simulink model "HILModel"  (Simulink 6.6)
settings: Solver=ode4  StartTime=0.0  StopTime=inf  FixedStep=SampleT  RelTol=1e-3
InitFcn:
  | clc
  | hilInit
values from neighbouring files (symbols this model uses):
  Euler_0 = [0; 0; 0*pi/180]'    [hilInit.m]
  HIL_K = 3    [hilInit.m]
  Pos_0 = [200; 350; 350]'    [hilInit.m]
  SampleT = 0.005    [hilInit.m]
  windBase = 3.5    [hilInit.m]
undefined symbols (not defined in the file or in its folder): A1, Apolar, bPWMda, bPWMde, bPWMdr, bPWMdt, CD0, chord, CL0, CLa, CLa_dot, Clb, ClDa, CLDe, CLDf, ClDr, clock, Clp, CLq, Clr, Cm0, Cma, CmDe, CmDf, Cmq, Cnb, CnDa, CnDr, Cnp, Cnr, CYb, CYDr, da_failamp, da_failbias, da_failper, daL_fail, daR_fail, DiscIntNeverNeededParam, dr_fail, Earth, elarm, F, GS_location, ISA_g, Ixx, Iyy, Izz, Light, mass, MIL, MinThK, mPWMda, mPWMde, mPWMdr, mPWMdt, PQR_0, span, tfailure, ThK, Vb_0 ... (+1)
libraries: simulink x31, aerolibconvert2 x8, xpclib x8, aerolibactuator x5, aerolibtransform2 x2, aerolibwind2 x2, dspmtrx3 x2, aerolibnav x2, aerolibatmos2 x1, aerolibanimutils x1
(part 1 of 2)
CloseFcn:
  | rtwprivate ssgencode ModelCloseRequest AttitudeComplementary
settings Model: Creator=ASL_Lab  LastModifiedBy=Administrator
settings DebuggingCC: AlgebraicLoopMsg=error  MultiTaskDSMMsg=warning  MultiTaskCondExecSysMsg=none  StrictBusMsg=None
settings HardwareCC: TargetHWDeviceType=32-bit Generic
settings RTWCC: IncludeERTFirstTime=on

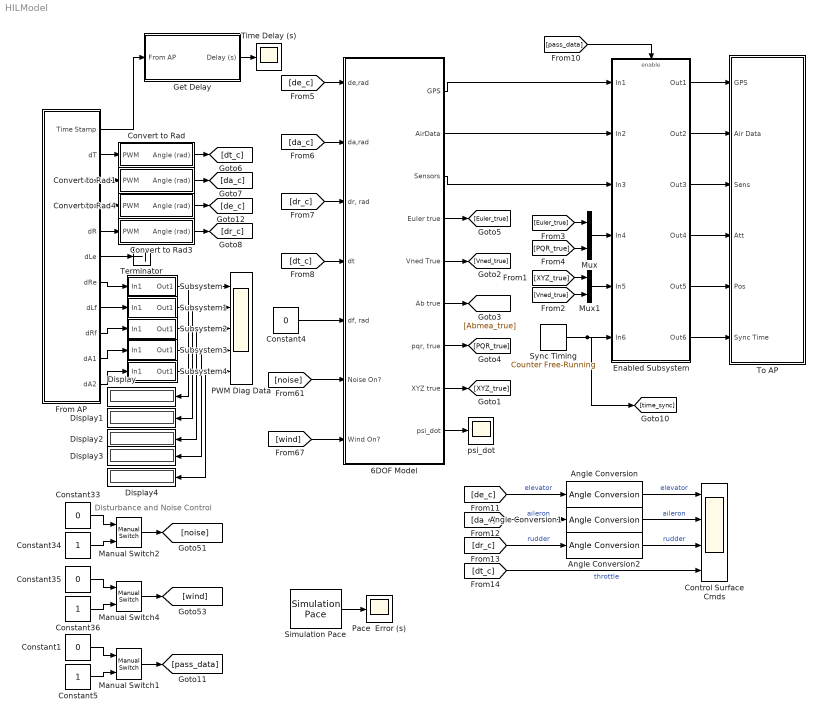
== system HILModel ==
  note: Disturbance and Noise Control
  6DOF Model : Subsystem
  Angle Conversion : aerolibconvert2/Angle Conversion  SystemSampleTime=-1  IU=rad  OU=deg
  Angle Conversion1 : aerolibconvert2/Angle Conversion  SystemSampleTime=-1  IU=rad  OU=deg
  Angle Conversion2 : aerolibconvert2/Angle Conversion  SystemSampleTime=-1  IU=rad  OU=deg
  Constant1 : Constant  Value=0  SampleTime=SampleT
  Constant33 : Constant  Value=0  SampleTime=SampleT
  Constant34 : Constant  SampleTime=SampleT
  Constant35 : Constant  Value=0  SampleTime=SampleT
  Constant36 : Constant  SampleTime=SampleT
  Constant4 : Constant  Value=0
  Constant5 : Constant  SampleTime=SampleT
  Control Surface Cmds : Scope  NumInputPorts=4
      settings: TimeRange=70  YMin=-55~-65~-75~-2.5  YMax=10~15~5~1  MaxDataPoints=25000
  Convert to Rad : Subsystem  mask{slopem=mPWMdt, interceptb=bPWMdt}
      mask prompts: slopem "Slope"; interceptb "Intercept"
  Convert to Rad1 : Subsystem  mask{slopem=mPWMda, interceptb=bPWMda}
      mask prompts: slopem "Slope"; interceptb "Intercept"
  Convert to Rad3 : Subsystem  mask{slopem=mPWMdr, interceptb=bPWMdr}
      mask prompts: slopem "Slope"; interceptb "Intercept"
  Convert to Rad4 : Subsystem  mask{slopem=mPWMde, interceptb=bPWMde}
      mask prompts: slopem "Slope"; interceptb "Intercept"
  Display{,1..4} (5 alike) : Display
  Enabled Subsystem : Subsystem  TreatAsAtomicUnit=on
  From AP : Subsystem
  Get Delay : Subsystem
  Manual Switch1 : simulink/Signal Routing/Manual Switch  SystemSampleTime=-1  sw=0  action=0  varsize=off
  Manual Switch2 : simulink/Signal Routing/Manual Switch  SystemSampleTime=-1  sw=1  action=0  varsize=off
  Manual Switch4 : simulink/Signal Routing/Manual Switch  SystemSampleTime=-1  sw=1  action=0  varsize=off
  Mux : Mux  Inputs=2
  Mux1 : Mux  Inputs=2
  PWM Diag Data : Scope  NumInputPorts=5
      settings: TimeRange=54.25925925925927  YMin=-31500~-33000~-34406.4~-34406.4~-35000  YMax=-28750~-28500~-31129.6~-31129.6~-15000  SaveName=ScopeData5  MaxDataPoints=25000
  Pace  Error (s) : Scope
      settings: YMin=-0.01  YMax=0.015  MaxDataPoints=25000
  Simulation Pace : aerolibanimutils/Simulation Pace  SimulationPace=1  SleepMode=MATLAB Thread  OutputPaceError=on  SampleTime=SampleT
      settings: AttributesFormatString=%<SimulationPace> sec/sec
  Subsystem : Subsystem
  Subsystem1 : Subsystem
  Subsystem2 : Subsystem
  Subsystem3 : Subsystem
  Subsystem4 : Subsystem
  Sync Timing : simulink/Sources/Counter Free-Running  SystemSampleTime=-1  NumBits=16  tsamp=SampleT
  Terminator : Terminator
  Time Delay (s) : Scope
      settings: TimeRange=60  YMin=0  YMax=0.05  SaveName=ScopeData2
  To AP : Subsystem
  psi_dot : Scope
      settings: TimeRange=120  YMin=-0.4  YMax=0.3  SaveName=ScopeData3  MaxDataPoints=25000
  wires:
  [PQR_true] -> Mux/2
  [XYZ_true] -> Mux1/1
  [Vned_true] -> Mux1/2
  [Euler_true] -> Mux/1
  Enabled Subsystem/1(Out1) -> To AP/1(GPS)
  Enabled Subsystem/2(Out2) -> To AP/2(Air Data)
  Enabled Subsystem/3(Out3) -> To AP/3(Sens)
  Enabled Subsystem/4(Out4) -> To AP/4(Att)
  Enabled Subsystem/5(Out5) -> To AP/5(Pos)
  Enabled Subsystem/6(Out6) -> To AP/6(Sync Time)
  6DOF Model/1(GPS) -> Enabled Subsystem/1(In1)
  6DOF Model/2(AirData) -> Enabled Subsystem/2(In2)
  6DOF Model/3(Sensors) -> Enabled Subsystem/3(In3)
  Mux/1 -> Enabled Subsystem/4(In4)
  Mux1/1 -> Enabled Subsystem/5(In5)
  Sync Timing/1 -> Enabled Subsystem/6(In6), [time_sync]
  6DOF Model/4(Euler true) -> [Euler_true]
  6DOF Model/5(Vned True) -> [Vned_true]
  6DOF Model/6(Ab true) -> [Abmea_true]
  6DOF Model/7("pqr, true") -> [PQR_true]
  6DOF Model/8(XYZ true) -> [XYZ_true]
  Constant4/1 -> 6DOF Model/5("df, rad")
  Constant33/1 -> Manual Switch2/1
  Constant34/1 -> Manual Switch2/2
  Manual Switch2/1 -> [noise]
  Constant35/1 -> Manual Switch4/1
  Constant36/1 -> Manual Switch4/2
  Manual Switch4/1 -> [wind]
  [noise] -> 6DOF Model/6(Noise On?)
  [wind] -> 6DOF Model/7(Wind On?)
  Constant1/1 -> Manual Switch1/1
  Constant5/1 -> Manual Switch1/2
  Manual Switch1/1 -> [pass_data]
  [pass_data] -> Enabled Subsystem/Enable
  From AP/3(dLa) -> Convert to Rad1/1(PWM)
  From AP/5(dR) -> Convert to Rad3/1(PWM)
  From AP/2(dT) -> Convert to Rad/1(PWM)
  From AP/4(dRa) -> Convert to Rad4/1(PWM)
  Get Delay/1(Delay (s)) -> Time Delay (s)/1
  From AP/1(Time Stamp) -> Get Delay/1(From AP)
  Convert to Rad/1(Angle (rad)) -> [dt_c]
  Convert to Rad1/1(Angle (rad)) -> [da_c]
  Convert to Rad3/1(Angle (rad)) -> [dr_c]
  From AP/6(dLe) -> Terminator/1
  [de_c] -> Angle Conversion/1  "elevator"
  [da_c] -> Angle Conversion1/1  "aileron"
  [dr_c] -> Angle Conversion2/1  "rudder"
  [dt_c] -> Control Surface Cmds/4  "throttle"
  [de_c] -> 6DOF Model/1(de,rad)
  [dt_c] -> 6DOF Model/4(dt)
  [dr_c] -> 6DOF Model/3("dr, rad")
  [da_c] -> 6DOF Model/2(da,rad)
  Angle Conversion/1 -> Control Surface Cmds/1  "elevator"
  Angle Conversion1/1 -> Control Surface Cmds/2  "aileron"
  Angle Conversion2/1 -> Control Surface Cmds/3  "rudder"
  Simulation Pace/1 -> Pace  Error (s)/1
  6DOF Model/9(psi_dot) -> psi_dot/1
  Subsystem/1(Out1) -> Display/1, PWM Diag Data/1
  Subsystem1/1(Out1) -> PWM Diag Data/2, Display1/1
  Subsystem2/1(Out1) -> PWM Diag Data/3, Display2/1
  Subsystem3/1(Out1) -> PWM Diag Data/4, Display3/1
  Subsystem4/1(Out1) -> PWM Diag Data/5, Display4/1
  From AP/7(dRe) -> Subsystem/1(In1)
  From AP/8(dLf) -> Subsystem1/1(In1)
  From AP/9(dRf) -> Subsystem2/1(In1)
  From AP/10(dA1) -> Subsystem3/1(In1)
  From AP/11(dA2) -> Subsystem4/1(In1)
  Convert to Rad4/1(Angle (rad)) -> [de_c]

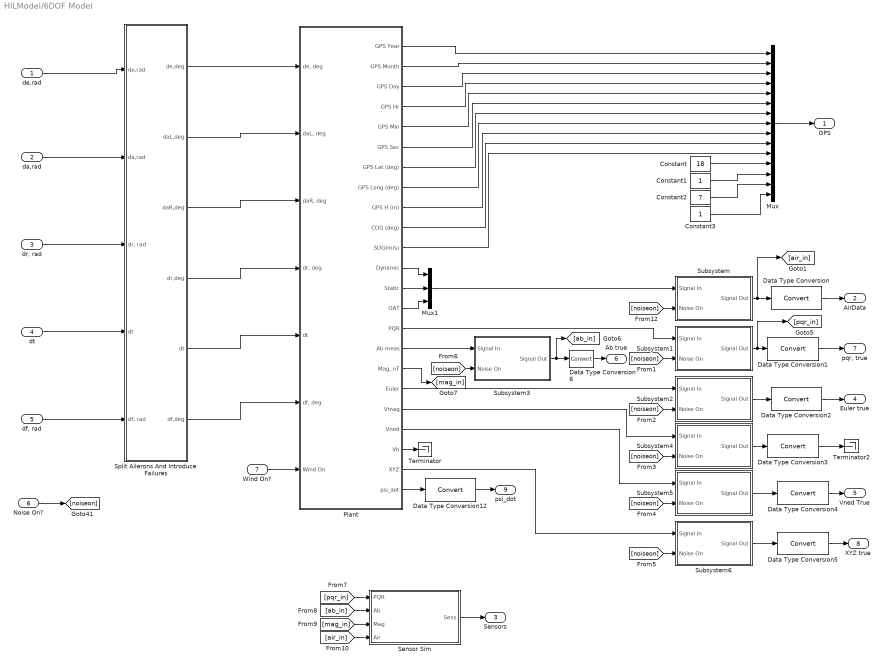
== system HILModel/6DOF Model ==
  de,rad : Inport
  da,rad : Inport  Port=2
  "dr, rad" : Inport  Port=3
  dt : Inport  Port=4
  "df, rad" : Inport  Port=5
  Noise On? : Inport  Port=6
  Wind On? : Inport  Port=7
  Constant : Constant  Value=18  SampleTime=SampleT
  Constant1 : Constant  SampleTime=SampleT
  Constant2 : Constant  Value=7  SampleTime=SampleT
  Constant3 : Constant  SampleTime=SampleT
  Data Type Conversion{,1..6,12} (8 alike) : DataTypeConversion  OutDataTypeMode=single
  Mux : Mux  Inputs=15
  Mux1 : Mux  Inputs=3
  Plant : Subsystem
  Sensor Sim : Subsystem
  Split Ailerons And Introduce Failures : Subsystem
  Subsystem : Subsystem  mask{nv=[0.01 0.01 0.1], st=SampleT, ns=[132 564 987]}
      mask prompts: nv "Noise Variance"; st "Sample Time"; ns "Noise Seed"
  Subsystem1 : Subsystem  mask{nv=[0.001 0.001 0.001], st=SampleT, ns=[132 564 987]}
      mask prompts: nv "Noise Variance"; st "Sample Time"; ns "Noise Seed"
  Subsystem2 : Subsystem  mask{nv=[0.0001 0.00003 0.0001], st=SampleT, ns=[132 564 987]}
      mask prompts: nv "Noise Variance"; st "Sample Time"; ns "Noise Seed"
  Subsystem3 : Subsystem  mask{nv=[0.1 0.1 0.1], st=SampleT, ns=[132 564 987]}
      mask prompts: nv "Noise Variance"; st "Sample Time"; ns "Noise Seed"
  Subsystem4 : Subsystem  mask{nv=[0.01], st=SampleT, ns=[321564]}
      mask prompts: nv "Noise Variance"; st "Sample Time"; ns "Noise Seed"
  Subsystem5 : Subsystem  mask{nv=[0.01 0.01 0.01], st=SampleT, ns=[321564 6546 98798]}
      mask prompts: nv "Noise Variance"; st "Sample Time"; ns "Noise Seed"
  Subsystem6 : Subsystem  mask{nv=[0.05 0.05 0.07], st=SampleT, ns=[321564]}
      mask prompts: nv "Noise Variance"; st "Sample Time"; ns "Noise Seed"
  Terminator : Terminator
  Terminator2 : Terminator
  GPS : Outport
  AirData : Outport  Port=2
  Sensors : Outport  Port=3
  Euler true : Outport  Port=4
  Vned True : Outport  Port=5
  Ab true : Outport  Port=6
  "pqr, true" : Outport  Port=7
  XYZ true : Outport  Port=8
  psi_dot : Outport  Port=9
  wires:
  Data Type Conversion12/1 -> psi_dot/1
  Data Type Conversion6/1 -> Ab true/1
  Data Type Conversion5/1 -> XYZ true/1
  Data Type Conversion4/1 -> Vned True/1
  Data Type Conversion3/1 -> Terminator2/1
  Data Type Conversion2/1 -> Euler true/1
  Data Type Conversion1/1 -> "pqr, true"/1
  Data Type Conversion/1 -> AirData/1
  Wind On?/1 -> Plant/7(Wind On)
  Plant/17("Mag, nT") -> [mag_in]
  Plant/21(Vb) -> Terminator/1
  Plant/22(XYZ) -> Subsystem6/1(Signal In)
  Subsystem6/1(Signal Out) -> Data Type Conversion5/1
  Plant/20(Vned) -> Subsystem5/1(Signal In)
  Subsystem5/1(Signal Out) -> Data Type Conversion4/1
  Plant/19(Vmag) -> Subsystem4/1(Signal In)
  Subsystem4/1(Signal Out) -> Data Type Conversion3/1
  Plant/16(Ab meas) -> Subsystem3/1(Signal In)
  Subsystem3/1(Signal Out) -> Data Type Conversion6/1, [ab_in]
  Plant/18(Euler) -> Subsystem2/1(Signal In)
  Subsystem2/1(Signal Out) -> Data Type Conversion2/1
  Plant/15(PQR) -> Subsystem1/1(Signal In)
  Subsystem1/1(Signal Out) -> Data Type Conversion1/1, [pqr_in]
  [noiseon] -> Subsystem3/2(Noise On)
  [noiseon] -> Subsystem6/2(Noise On)
  [noiseon] -> Subsystem5/2(Noise On)
  [noiseon] -> Subsystem4/2(Noise On)
  [noiseon] -> Subsystem2/2(Noise On)
  [noiseon] -> Subsystem1/2(Noise On)
  [noiseon] -> Subsystem/2(Noise On)
  Subsystem/1(Signal Out) -> Data Type Conversion/1, [air_in]
  Noise On?/1 -> [noiseon]
  Plant/23(psi_dot) -> Data Type Conversion12/1
  Constant3/1 -> Mux/15
  Constant2/1 -> Mux/14
  Constant1/1 -> Mux/13
  Constant/1 -> Mux/12
  Mux1/1 -> Subsystem/1(Signal In)
  Plant/14(OAT) -> Mux1/3
  Plant/13(Static) -> Mux1/2
  Plant/12(Dynamic) -> Mux1/1
  Plant/11(SOG(m/s)) -> Mux/11
  Plant/10(COG (deg)) -> Mux/10
  Plant/9(GPS H (m)) -> Mux/9
  Plant/8(GPS Long (deg)) -> Mux/8
  Plant/7(GPS Lat (deg)) -> Mux/7
  Plant/6(GPS Sec) -> Mux/6
  Plant/5(GPS Min) -> Mux/5
  Plant/4(GPS Hr) -> Mux/4
  Plant/3(GPS Day) -> Mux/3
  Plant/2(GPS Month) -> Mux/2
  Plant/1(GPS Year) -> Mux/1
  Mux/1 -> GPS/1
  "df, rad"/1 -> Split Ailerons And Introduce Failures/5("df, rad")
  dt/1 -> Split Ailerons And Introduce Failures/4(dt)
  "dr, rad"/1 -> Split Ailerons And Introduce Failures/3("dr, rad")
  da,rad/1 -> Split Ailerons And Introduce Failures/2(da,rad)
  de,rad/1 -> Split Ailerons And Introduce Failures/1(de,rad)
  Sensor Sim/1(Sens) -> Sensors/1
  [pqr_in] -> Sensor Sim/1(PQR)
  [ab_in] -> Sensor Sim/2(Ab)
  [mag_in] -> Sensor Sim/3(Mag)
  Split Ailerons And Introduce Failures/1(de,deg) -> Plant/1("de, deg")
  Split Ailerons And Introduce Failures/2(daL,deg) -> Plant/2("daL, deg")
  Split Ailerons And Introduce Failures/3(daR,deg) -> Plant/3("daR, deg")
  Split Ailerons And Introduce Failures/4(dr,deg) -> Plant/4("dr, deg")
  Split Ailerons And Introduce Failures/5("dt ") -> Plant/5(dt)
  Split Ailerons And Introduce Failures/6(df,deg) -> Plant/6("df, deg")
  [air_in] -> Sensor Sim/4(Air)

== system HILModel/Convert to Rad ==
  PWM : Inport  Orientation=down
  Add : Sum  OutScaling=2^-10
  Constant1 : Constant  Value=slopem
  Constant2 : Constant  Value=interceptb
  Data Type Conversion : DataTypeConversion  OutDataTypeMode=single
  Divide : Product  OutScaling=2^-10
  Angle (rad) : Outport
  wires:
  Constant1/1 -> Divide/2
  Add/1 -> Data Type Conversion/1
  Divide/1 -> Add/1
  Constant2/1 -> Add/2
  PWM/1 -> Divide/1
  Data Type Conversion/1 -> Angle (rad)/1

== system HILModel/Convert to Rad1 ==
  PWM : Inport  Orientation=down
  Add : Sum  OutScaling=2^-10
  Constant1 : Constant  Value=slopem
  Constant2 : Constant  Value=interceptb
  Data Type Conversion : DataTypeConversion  OutDataTypeMode=single
  Divide : Product  OutScaling=2^-10
  Angle (rad) : Outport
  wires:
  Data Type Conversion/1 -> Angle (rad)/1
  PWM/1 -> Divide/1
  Constant2/1 -> Add/2
  Divide/1 -> Add/1
  Add/1 -> Data Type Conversion/1
  Constant1/1 -> Divide/2

== system HILModel/Convert to Rad3 ==
  PWM : Inport  Orientation=down
  Add : Sum  OutScaling=2^-10
  Constant1 : Constant  Value=slopem
  Constant2 : Constant  Value=interceptb
  Data Type Conversion : DataTypeConversion  OutDataTypeMode=single
  Divide : Product  OutScaling=2^-10
  Angle (rad) : Outport
  wires:
  Data Type Conversion/1 -> Angle (rad)/1
  PWM/1 -> Divide/1
  Constant2/1 -> Add/2
  Divide/1 -> Add/1
  Add/1 -> Data Type Conversion/1
  Constant1/1 -> Divide/2

== system HILModel/Convert to Rad4 ==
  PWM : Inport  Orientation=down
  Add : Sum  OutScaling=2^-10
  Constant1 : Constant  Value=slopem
  Constant2 : Constant  Value=interceptb
  Data Type Conversion : DataTypeConversion  OutDataTypeMode=single
  Divide : Product  OutScaling=2^-10
  Angle (rad) : Outport
  wires:
  Data Type Conversion/1 -> Angle (rad)/1
  PWM/1 -> Divide/1
  Constant2/1 -> Add/2
  Divide/1 -> Add/1
  Add/1 -> Data Type Conversion/1
  Constant1/1 -> Divide/2

== system HILModel/Enabled Subsystem ==
  In1 : Inport
  In2 : Inport  Port=2
  In3 : Inport  Port=3
  In4 : Inport  Port=4
  In5 : Inport  Port=5
  In6 : Inport  Port=6
  Enable : EnablePort
  Out1 : Outport
  Out2 : Outport  Port=2
  Out3 : Outport  Port=3
  Out4 : Outport  Port=4
  Out5 : Outport  Port=5
  Out6 : Outport  Port=6
  wires:
  In1/1 -> Out1/1
  In2/1 -> Out2/1
  In3/1 -> Out3/1
  In4/1 -> Out4/1
  In5/1 -> Out5/1
  In6/1 -> Out6/1

== system HILModel/From AP ==
  Bus Creator : BusCreator  Inputs=11
  Bus Selector : BusSelector  OutputSignals=dt,dla,dra,dr,dle,dre,dlf,drf,da1,da2,timeStamp
  Display : Display
  Receive : xpclib/UDP/Receive  ipAddress=0.0.0.0  ipPort=5678  width=22  sampletime=SampleT
  Terminator : Terminator
  Unpack1 : xpclib/UDP/Unpack  dimensions={1,1,1,1,1,1,1,1,1,1,1}  datatypes={'uint16','uint16','uint16','uint16', 'uint16', 'uint16','uint16', 'uint16','uint16', 'uint16','uint16'}  byteAlign=1
  Time Stamp : Outport
  dT : Outport  Port=2
  dLa : Outport  Port=3
  dRa : Outport  Port=4
  dR : Outport  Port=5
  dLe : Outport  Port=6
  dRe : Outport  Port=7
  dLf : Outport  Port=8
  dRf : Outport  Port=9
  dA1 : Outport  Port=10
  dA2 : Outport  Port=11
  wires:
  Receive/1 -> Unpack1/1
  Receive/2 -> Terminator/1
  Bus Creator/1 -> Bus Selector/1, Display/1
  Unpack1/1 -> Bus Creator/1  "dt"
  Unpack1/3 -> Bus Creator/3  "dra"
  Unpack1/5 -> Bus Creator/5  "dle"
  Unpack1/7 -> Bus Creator/7  "dlf"
  Unpack1/9 -> Bus Creator/9  "da1"
  Unpack1/11 -> Bus Creator/11  "timeStamp"
  Bus Selector/1 -> dT/1  "<dt>"
  Bus Selector/2 -> dLa/1  "<dla>"
  Bus Selector/3 -> dRa/1  "<dra>"
  Bus Selector/4 -> dR/1  "<dr>"
  Bus Selector/5 -> dLe/1  "<dle>"
  Bus Selector/6 -> dRe/1  "<dre>"
  Bus Selector/7 -> dLf/1  "<dlf>"
  Bus Selector/8 -> dRf/1  "<drf>"
  Bus Selector/9 -> dA1/1  "<da1>"
  Bus Selector/10 -> dA2/1  "<da2>"
  Bus Selector/11 -> Time Stamp/1  "<timeStamp>"
  Unpack1/2 -> Bus Creator/2  "dla"
  Unpack1/4 -> Bus Creator/4  "dr"
  Unpack1/6 -> Bus Creator/6  "dre"
  Unpack1/8 -> Bus Creator/8  "drf"
  Unpack1/10 -> Bus Creator/10  "da2"

== system HILModel/Get Delay ==
  From AP : Inport
  Detect Change : Subsystem
  GPSAlive : Subsystem
  Delay (s) : Outport
  wires:
  From AP/1 -> Detect Change/1(Data)
  Detect Change/1(change?) -> GPSAlive/1(update?)
  GPSAlive/1(Update TIme) -> Delay (s)/1

== system HILModel/Subsystem ==
  In1 : Inport
  Add : Sum  Inputs=+-  OutScaling=2^-10
  Constant : Constant  Value=32768
  Out1 : Outport
  wires:
  Constant/1 -> Add/2
  In1/1 -> Add/1
  Add/1 -> Out1/1

== system HILModel/Subsystem1 ==
  In1 : Inport
  Add : Sum  Inputs=+-  OutScaling=2^-10
  Constant : Constant  Value=32768
  Out1 : Outport
  wires:
  Add/1 -> Out1/1
  In1/1 -> Add/1
  Constant/1 -> Add/2

== system HILModel/Subsystem2 ==
  In1 : Inport
  Add : Sum  Inputs=+-  OutScaling=2^-10
  Constant : Constant  Value=32768
  Out1 : Outport
  wires:
  Constant/1 -> Add/2
  In1/1 -> Add/1
  Add/1 -> Out1/1

== system HILModel/Subsystem3 ==
  In1 : Inport
  Add : Sum  Inputs=+-  OutScaling=2^-10
  Constant : Constant  Value=32768
  Out1 : Outport
  wires:
  Add/1 -> Out1/1
  In1/1 -> Add/1
  Constant/1 -> Add/2

== system HILModel/Subsystem4 ==
  In1 : Inport
  Add : Sum  Inputs=+-  OutScaling=2^-10
  Constant : Constant  Value=32768
  Out1 : Outport
  wires:
  Constant/1 -> Add/2
  In1/1 -> Add/1
  Add/1 -> Out1/1

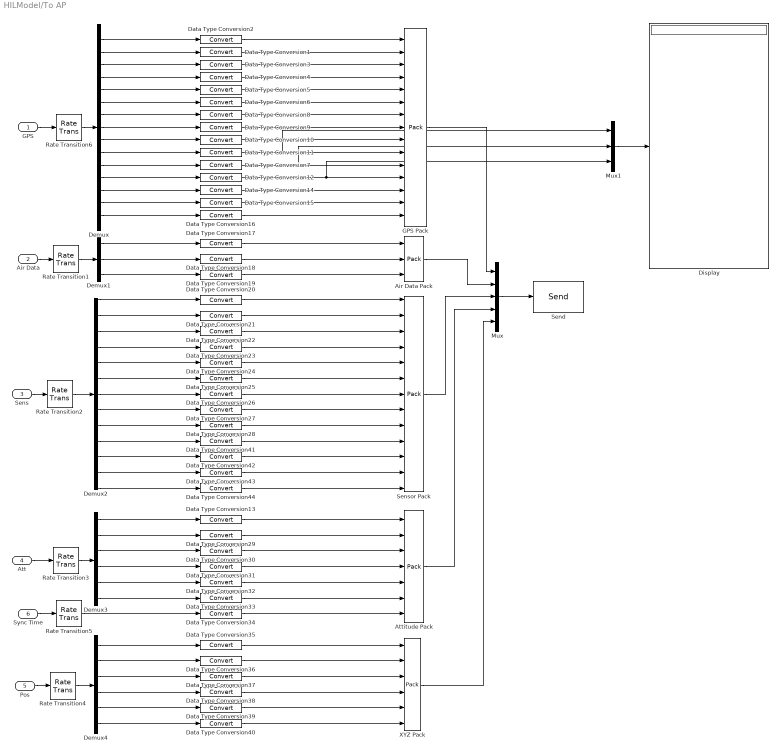
== system HILModel/To AP ==
  GPS : Inport
  Air Data : Inport  Port=2
  Sens : Inport  Port=3
  Att : Inport  Port=4
  Pos : Inport  Port=5
  Sync Time : Inport  Port=6
  Air Data Pack : xpclib/UDP/Pack  datatypes={'single', 'single', 'int16'}  byteAlign=1
  Attitude Pack : xpclib/UDP/Pack  datatypes={'single','single','single','single','single','single','uint16'}  byteAlign=1
  Data Type Conversion{1..6,14..16} (9 alike) : DataTypeConversion  OutDataTypeMode=uint8
  Data Type Conversion{8..10,13,17..18,29..33,35..40} (17 alike) : DataTypeConversion  OutDataTypeMode=single
  Data Type Conversion{7,11..12,34} (4 alike) : DataTypeConversion  OutDataTypeMode=uint16
  Data Type Conversion{19..28,41..44} (14 alike) : DataTypeConversion  OutDataTypeMode=int16
  Demux : Demux  Outputs=15
  Demux1 : Demux  Outputs=3
  Demux2 : Demux  Outputs=13
  Demux3 : Demux  Outputs=6
  Demux4 : Demux  Outputs=6
  Display : Display
  GPS Pack : xpclib/UDP/Pack  datatypes={'uint8','uint8','uint8','uint8','uint8','uint8', 'single', 'single', 'single', 'uint16', 'uint16', 'uint16', 'uint8', 'uint8', 'uint8'}  byteAlign=1
  Mux : Mux  Inputs=5
  Mux1 : Mux  Inputs=3
  Rate Transition{1..6} (6 alike) : RateTransition  OutPortSampleTime=SampleT*HIL_K
  Send : xpclib/UDP/Send  ipAddress=255.255.255.255  ipPort=5679  localPort=5678  sampletime=SampleT*HIL_K
  Sensor Pack : xpclib/UDP/Pack  datatypes={'int16', 'int16', 'int16', 'int16', 'int16', 'int16', 'int16', 'int16', 'int16', 'int16', 'int16', 'int16', 'int16'}  byteAlign=1
  XYZ Pack : xpclib/UDP/Pack  datatypes={'single','single','single','single','single','single'}  byteAlign=1
  wires:
  Demux/1 -> Data Type Conversion2/1
  Demux/2 -> Data Type Conversion1/1
  Demux/3 -> Data Type Conversion3/1
  Demux/4 -> Data Type Conversion4/1
  Demux/5 -> Data Type Conversion5/1
  Demux/6 -> Data Type Conversion6/1
  Demux/7 -> Data Type Conversion8/1
  Demux/8 -> Data Type Conversion9/1
  Demux/9 -> Data Type Conversion10/1
  Demux/10 -> Data Type Conversion11/1
  Demux/11 -> Data Type Conversion7/1
  Demux/12 -> Data Type Conversion12/1
  Demux/13 -> Data Type Conversion14/1
  Demux/14 -> Data Type Conversion15/1
  Demux/15 -> Data Type Conversion16/1
  Demux1/2 -> Data Type Conversion18/1
  Demux1/3 -> Data Type Conversion19/1
  Demux2/1 -> Data Type Conversion20/1
  Demux2/2 -> Data Type Conversion21/1
  Demux2/3 -> Data Type Conversion22/1
  Demux2/4 -> Data Type Conversion23/1
  Demux2/5 -> Data Type Conversion24/1
  Demux2/6 -> Data Type Conversion25/1
  Demux2/7 -> Data Type Conversion26/1
  Demux2/8 -> Data Type Conversion27/1
  Demux2/9 -> Data Type Conversion28/1
  Mux/1 -> Send/1
  GPS Pack/1 -> Mux/1
  Air Data Pack/1 -> Mux/2
  Sensor Pack/1 -> Mux/3
  GPS/1 -> Rate Transition6/1
  Air Data/1 -> Rate Transition1/1
  Sens/1 -> Rate Transition2/1
  Rate Transition6/1 -> Demux/1
  Rate Transition1/1 -> Demux1/1
  Rate Transition2/1 -> Demux2/1
  Att/1 -> Rate Transition3/1
  Pos/1 -> Rate Transition4/1
  Rate Transition3/1 -> Demux3/1
  Demux3/1 -> Data Type Conversion13/1
  Demux3/2 -> Data Type Conversion29/1
  Demux3/3 -> Data Type Conversion30/1
  Demux3/4 -> Data Type Conversion31/1
  Demux3/5 -> Data Type Conversion32/1
  Demux3/6 -> Data Type Conversion33/1
  Demux4/1 -> Data Type Conversion35/1
  Demux4/2 -> Data Type Conversion36/1
  Demux4/3 -> Data Type Conversion37/1
  Demux4/4 -> Data Type Conversion38/1
  Demux4/5 -> Data Type Conversion39/1
  Demux4/6 -> Data Type Conversion40/1
  Rate Transition4/1 -> Demux4/1
  Attitude Pack/1 -> Mux/4
  XYZ Pack/1 -> Mux/5
  Sync Time/1 -> Rate Transition5/1
  Data Type Conversion2/1 -> GPS Pack/1
  Data Type Conversion1/1 -> GPS Pack/2
  Data Type Conversion3/1 -> GPS Pack/3
  Data Type Conversion4/1 -> GPS Pack/4
  Data Type Conversion5/1 -> GPS Pack/5
  Data Type Conversion6/1 -> GPS Pack/6
  Data Type Conversion8/1 -> GPS Pack/7
  Data Type Conversion9/1 -> GPS Pack/8
  Data Type Conversion10/1 -> GPS Pack/9
  Data Type Conversion11/1 -> GPS Pack/10, Mux1/1
  Data Type Conversion7/1 -> GPS Pack/11, Mux1/2
  Data Type Conversion12/1 -> GPS Pack/12, Mux1/3
  Data Type Conversion14/1 -> GPS Pack/13
  Data Type Conversion15/1 -> GPS Pack/14
  Data Type Conversion16/1 -> GPS Pack/15
  Data Type Conversion17/1 -> Air Data Pack/1
  Data Type Conversion18/1 -> Air Data Pack/2
  Data Type Conversion19/1 -> Air Data Pack/3
  Data Type Conversion20/1 -> Sensor Pack/1
  Data Type Conversion21/1 -> Sensor Pack/2
  Data Type Conversion22/1 -> Sensor Pack/3
  Data Type Conversion23/1 -> Sensor Pack/4
  Data Type Conversion24/1 -> Sensor Pack/5
  Data Type Conversion25/1 -> Sensor Pack/6
  Data Type Conversion26/1 -> Sensor Pack/7
  Data Type Conversion27/1 -> Sensor Pack/8
  Data Type Conversion28/1 -> Sensor Pack/9
  Data Type Conversion13/1 -> Attitude Pack/1
  Data Type Conversion29/1 -> Attitude Pack/2
  Data Type Conversion30/1 -> Attitude Pack/3
  Data Type Conversion31/1 -> Attitude Pack/4
  Data Type Conversion32/1 -> Attitude Pack/5
  Data Type Conversion33/1 -> Attitude Pack/6
  Data Type Conversion34/1 -> Attitude Pack/7
  Data Type Conversion35/1 -> XYZ Pack/1
  Data Type Conversion36/1 -> XYZ Pack/2
  Data Type Conversion37/1 -> XYZ Pack/3
  Data Type Conversion38/1 -> XYZ Pack/4
  Data Type Conversion39/1 -> XYZ Pack/5
  Data Type Conversion40/1 -> XYZ Pack/6
  Demux1/1 -> Data Type Conversion17/1
  Rate Transition5/1 -> Data Type Conversion34/1
  Demux2/10 -> Data Type Conversion41/1
  Data Type Conversion41/1 -> Sensor Pack/10
  Demux2/11 -> Data Type Conversion42/1
  Data Type Conversion42/1 -> Sensor Pack/11
  Demux2/12 -> Data Type Conversion43/1
  Data Type Conversion43/1 -> Sensor Pack/12
  Demux2/13 -> Data Type Conversion44/1
  Data Type Conversion44/1 -> Sensor Pack/13
  Mux1/1 -> Display/1

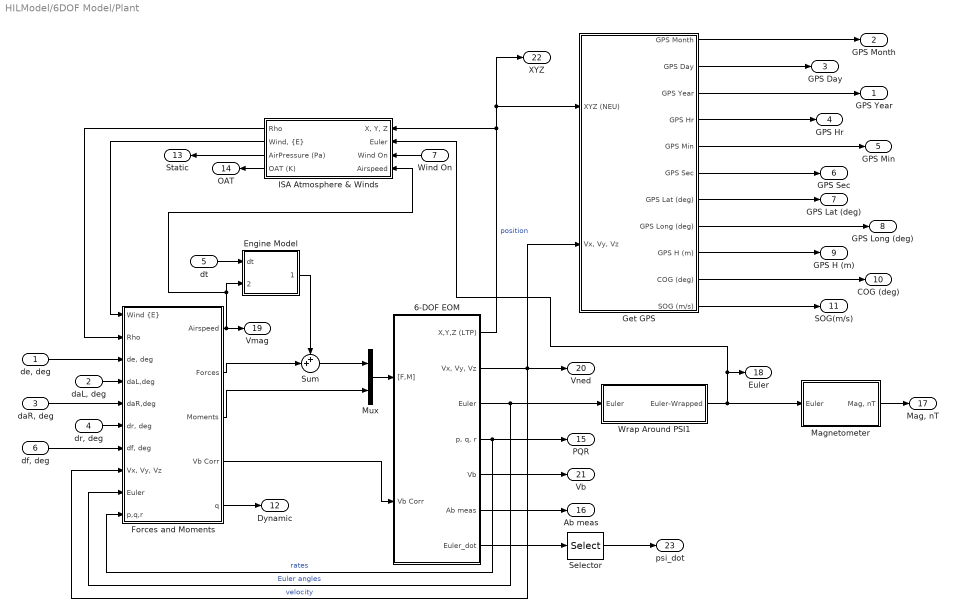
== system HILModel/6DOF Model/Plant ==
  "de, deg" : Inport
  "daL, deg" : Inport  Port=2
  "daR, deg" : Inport  Port=3
  "dr, deg" : Inport  Port=4
  dt : Inport  Port=5
  "df, deg" : Inport  Port=6
  Wind On : Inport  Orientation=left  Port=7
  6-DOF EOM : Subsystem
  Engine Model : Subsystem
  Forces and Moments : Subsystem
  Get GPS : Subsystem
  ISA Atmosphere & Winds : Subsystem  Orientation=left
  Magnetometer : Subsystem  mask{magField=[ 23143.6 5858.2 45511.9]}
      mask prompts: magField "Local Magnetic Field"
      mask help:
      | Simulates the Data from magnetometers with no noise.
      |
      | You can obtain data for the local magnetic field at:
      |
      | http://www.ngdc.noaa.gov/geomagmodels/IGRFWMM.jsp
  Mux : Mux  Inputs=2
  Selector : Selector  IndexOptions=Index vector (dialog)  Indices=[3]  OutputSizes=1  InputPortWidth=3
  Sum : Sum  Inputs=++|  SaturateOnIntegerOverflow=on
  Wrap Around PSI1 : Subsystem
  GPS Year : Outport
  GPS Month : Outport  Port=2
  GPS Day : Outport  Port=3
  GPS Hr : Outport  Port=4
  GPS Min : Outport  Port=5
  GPS Sec : Outport  Port=6
  GPS Lat (deg) : Outport  Port=7
  GPS Long (deg) : Outport  Port=8
  GPS H (m) : Outport  Port=9
  COG (deg) : Outport  Port=10
  SOG(m/s) : Outport  Port=11
  Dynamic : Outport  Port=12
  Static : Outport  Orientation=left  Port=13
  OAT : Outport  Orientation=left  Port=14
  PQR : Outport  Port=15
  Ab meas : Outport  Port=16
  "Mag, nT" : Outport  Port=17
  Euler : Outport  Port=18
  Vmag : Outport  Port=19
  Vned : Outport  Port=20
  Vb : Outport  Port=21
  XYZ : Outport  Port=22
  psi_dot : Outport  Port=23
  wires:
  Get GPS/1(GPS Month) -> GPS Month/1
  Get GPS/2(GPS Day) -> GPS Day/1
  Get GPS/3(GPS Year) -> GPS Year/1
  Get GPS/4(GPS Hr) -> GPS Hr/1
  Get GPS/5(GPS Min) -> GPS Min/1
  Get GPS/6(GPS Sec) -> GPS Sec/1
  Get GPS/7(GPS Lat (deg)) -> GPS Lat (deg)/1
  Get GPS/8(GPS Long (deg)) -> GPS Long (deg)/1
  Get GPS/9(GPS H (m)) -> GPS H (m)/1
  6-DOF EOM/6(Ab meas) -> Ab meas/1
  Mux/1 -> 6-DOF EOM/1("[F,M]")
  6-DOF EOM/5(Vb) -> Vb/1
  Engine Model/1(Thrust) -> Sum/1
  Forces and Moments/5(q) -> Dynamic/1
  ISA Atmosphere & Winds/3(AirPressure (Pa)) -> Static/1
  Forces and Moments/1(Airspeed) -> Vmag/1, Engine Model/2(Vmag), ISA Atmosphere & Winds/4(Airspeed)
  ISA Atmosphere & Winds/2("Wind, {E}") -> Forces and Moments/1("Wind {E}")
  ISA Atmosphere & Winds/1(Rho) -> Forces and Moments/2(Rho)
  Forces and Moments/3(Moments) -> Mux/2
  Forces and Moments/2(Forces) -> Sum/2
  Sum/1 -> Mux/1
  Forces and Moments/4(Vb Corr) -> 6-DOF EOM/2(Vb Corr)
  6-DOF EOM/1(X,Y,Z (LTP)) -> ISA Atmosphere & Winds/1("X, Y, Z"), Get GPS/1(XYZ (NEU)), XYZ/1  "position"
  6-DOF EOM/2("Vx, Vy, Vz") -> Vned/1, Get GPS/2("Vx, Vy, Vz"), Forces and Moments/8("Vx, Vy, Vz ")  "velocity"
  6-DOF EOM/3(Euler) -> Wrap Around PSI1/1(Euler), Forces and Moments/9(Euler)  "Euler angles"
  6-DOF EOM/4("p, q, r") -> PQR/1, Forces and Moments/10(p,q,r)  "rates"
  dt/1 -> Engine Model/1(dt)
  "de, deg"/1 -> Forces and Moments/3("de, deg")
  "daL, deg"/1 -> Forces and Moments/4(daL,deg)
  "dr, deg"/1 -> Forces and Moments/6("dr, deg")
  "df, deg"/1 -> Forces and Moments/7("df, deg")
  Wrap Around PSI1/1(Euler-Wrapped) -> Magnetometer/1(Euler), Euler/1, ISA Atmosphere & Winds/2(Euler)
  Magnetometer/1("Mag, nT") -> "Mag, nT"/1
  Get GPS/10(COG (deg)) -> COG (deg)/1
  Get GPS/11(SOG (m/s)) -> SOG(m/s)/1
  ISA Atmosphere & Winds/4(OAT (K)) -> OAT/1
  6-DOF EOM/7(Euler_dot) -> Selector/1
  Selector/1 -> psi_dot/1
  Wind On/1 -> ISA Atmosphere & Winds/3(Wind On)
  "daR, deg"/1 -> Forces and Moments/5(daR,deg)

== system HILModel/6DOF Model/Sensor Sim ==
  PQR : Inport
  Ab : Inport  Port=2
  Mag : Inport  Port=3
  Air : Inport  Port=4
  Constant : Constant  Value=2048
  Mux1 : Mux  Inputs=3
  Mux2 : Mux
  Selector : Selector  IndexOptions=Index vector (dialog)  Indices=[2 1]  OutputSizes=1  InputPortWidth=3
  Selector1 : Selector  IndexOptions=Index vector (dialog)  Indices=[3]  OutputSizes=1  InputPortWidth=3
  Three-axis Accelerometer : aerolibnav/Three-axis Accelerometer  SystemSampleTime=-1  units=Metric (MKS)  acc=[0 0 0]  gtype=off  dtype_a=on  w_a=190  z_a=0.707  a_sf_cc=[-41 0 0; 0 41 0; 0 0 -43]  a_bias=[2015 2018 2006]  a_rand=off  a_seeds=[23093 23094 23095]  a_pow=[0.008 0.008 0.008]  a_sat="[-inf  -inf  -inf  inf inf inf]"  a_Ts=SampleT
  Three-axis Gyroscope : aerolibnav/Three-axis Gyroscope  SystemSampleTime=-1  dtype_g=off  w_g=190  z_g=0.707  g_sf_cc=[-142 0 0; 0 142 0; 0 0 235]  g_bias=[1866 1981 2042]  g_sen=[0 0 0]  g_rand=off  g_seeds=[23093 23094 23095]  g_pow=[0.008 0.008 0.008]  g_sat="[-inf  -inf  -inf  inf inf inf]"  g_Ts=SampleT
  Sens : Outport
  wires:
  Mag/1 -> Mux2/3
  Mux2/1 -> Sens/1
  Ab/1 -> Three-axis Accelerometer/1
  PQR/1 -> Three-axis Gyroscope/1
  Three-axis Accelerometer/1 -> Mux2/2
  Three-axis Gyroscope/1 -> Mux2/1
  Air/1 -> Selector/1, Selector1/1
  Selector/1 -> Mux1/1
  Constant/1 -> Mux1/2
  Selector1/1 -> Mux1/3
  Mux1/1 -> Mux2/4

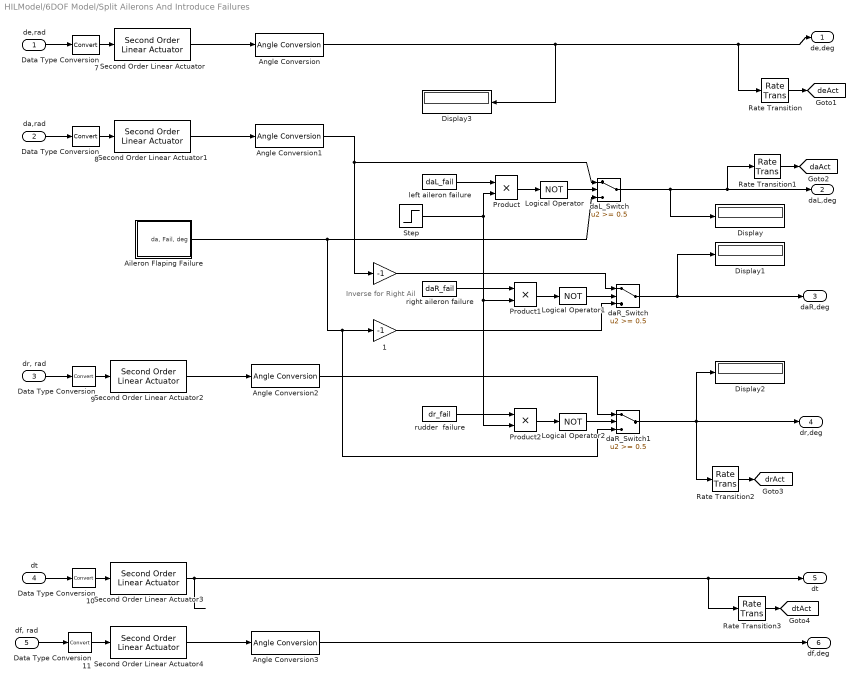
== system HILModel/6DOF Model/Split Ailerons And Introduce Failures ==
  note: Inverse
      | for Right
      | Ail
  de,rad : Inport
  da,rad : Inport  Port=2
  "dr, rad" : Inport  Port=3
  dt : Inport  Port=4
  "df, rad" : Inport  Port=5
  " " : Gain  Gain=-1  SaturateOnIntegerOverflow=on
  " 1" : Gain  Gain=-1  SaturateOnIntegerOverflow=on
  Aileron Flaping Failure : Subsystem
  Angle Conversion{,1..3} (4 alike) : aerolibconvert2/Angle Conversion  SystemSampleTime=-1  IU=rad  OU=deg
  Data Type Conversion{7..11} (5 alike) : DataTypeConversion  OutDataTypeMode=double
  Display{,1..3} (4 alike) : Display
  Logical Operator : Logic  Operator=NOT  AllPortsSameDT=off  OutDataTypeMode=Boolean
  Logical Operator1 : Logic  Operator=NOT  AllPortsSameDT=off  OutDataTypeMode=Boolean
  Logical Operator2 : Logic  Operator=NOT  AllPortsSameDT=off  OutDataTypeMode=Boolean
  Product : Product  RndMeth=Zero
  Product1 : Product  RndMeth=Zero
  Product2 : Product  RndMeth=Zero
  Rate Transition{,1..3} (4 alike) : RateTransition  OutPortSampleTime=apSampleTime
  Second Order Linear Actuator{,1..3} (4 alike) : aerolibactuator/Second Order Linear Actuator  SystemSampleTime=-1  wn_fin=15  z_fin=0.8  fin_act_0=0
  Second Order Linear Actuator4 : aerolibactuator/Second Order Linear Actuator  SystemSampleTime=-1  wn_fin=150  z_fin=0.7  fin_act_0=0
  Step : Step  Time=tfailure
  daL_Switch : Switch  Threshold=0.5
  daR_Switch : Switch  Threshold=0.5
  daR_Switch1 : Switch  Threshold=0.5
  left aileron failure : Constant  Value=daL_fail
  right aileron failure : Constant  Value=daR_fail
  rudder  failure : Constant  Value=dr_fail
  de,deg : Outport
  daL,deg : Outport  Port=2
  daR,deg : Outport  Port=3
  dr,deg : Outport  Port=4
  "dt " : Outport  Port=5
  df,deg : Outport  Port=6
  tag scope: daAct=global, deAct=global, drAct=global, dtAct=global
  wires:
  Rate Transition/1 -> [deAct]
  daR_Switch1/1 -> Rate Transition2/1, Display2/1, dr,deg/1
  Logical Operator2/1 -> daR_Switch1/2
  Product2/1 -> Logical Operator2/1
  rudder  failure/1 -> Product2/1
  daR_Switch/1 -> Display1/1, daR,deg/1
  " 1"/1 -> daR_Switch/3
  " "/1 -> daR_Switch/1
  Logical Operator1/1 -> daR_Switch/2
  Product1/1 -> Logical Operator1/1
  right aileron failure/1 -> Product1/1
  daL_Switch/1 -> Rate Transition1/1, daL,deg/1, Display/1
  Step/1 -> Product2/2, Product1/2, Product/2
  Logical Operator/1 -> daL_Switch/2
  Product/1 -> Logical Operator/1
  Aileron Flaping Failure/1("da, Fail, deg") -> daR_Switch1/3, " 1"/1, daL_Switch/3
  left aileron failure/1 -> Product/1
  Angle Conversion3/1 -> df,deg/1
  Angle Conversion2/1 -> daR_Switch1/1
  Angle Conversion1/1 -> " "/1, daL_Switch/1
  Angle Conversion/1 -> Rate Transition/1, de,deg/1, Display3/1
  Data Type Conversion11/1 -> Second Order Linear Actuator4/1
  Data Type Conversion10/1 -> Second Order Linear Actuator3/1
  Data Type Conversion9/1 -> Second Order Linear Actuator2/1
  Data Type Conversion8/1 -> Second Order Linear Actuator1/1
  Data Type Conversion7/1 -> Second Order Linear Actuator/1
  Rate Transition3/1 -> [dtAct]
  Rate Transition2/1 -> [drAct]
  Rate Transition1/1 -> [daAct]
  Second Order Linear Actuator4/1 -> Angle Conversion3/1
  Second Order Linear Actuator3/1 -> Rate Transition3/1, "dt "/1
  Second Order Linear Actuator2/1 -> Angle Conversion2/1
  Second Order Linear Actuator1/1 -> Angle Conversion1/1
  Second Order Linear Actuator/1 -> Angle Conversion/1
  "df, rad"/1 -> Data Type Conversion11/1
  dt/1 -> Data Type Conversion10/1
  "dr, rad"/1 -> Data Type Conversion9/1
  da,rad/1 -> Data Type Conversion8/1
  de,rad/1 -> Data Type Conversion7/1

== system HILModel/6DOF Model/Subsystem ==
  Signal In : Inport  Orientation=down
  Noise On : Inport  Port=2
  Add : Sum  OutScaling=2^-10
  Random Number : RandomNumber  Variance=nv  Seed=ns  SampleTime=st
  Signal1 : InportShadow  Port=1  LatchByCopyingInsideSignal=off
  Switch : Switch  Threshold=0.3
  Signal Out : Outport
  wires:
  Signal1/1 -> Switch/3
  Switch/1 -> Signal Out/1
  Noise On/1 -> Switch/2
  Signal In/1 -> Add/1
  Add/1 -> Switch/1
  Random Number/1 -> Add/2

== system HILModel/6DOF Model/Subsystem1 ==
  Signal In : Inport  Orientation=down
  Noise On : Inport  Port=2
  Add : Sum  OutScaling=2^-10
  Random Number : RandomNumber  Variance=nv  Seed=ns  SampleTime=st
  Signal1 : InportShadow  Port=1  LatchByCopyingInsideSignal=off
  Switch : Switch  Threshold=0.3
  Signal Out : Outport
  wires:
  Random Number/1 -> Add/2
  Add/1 -> Switch/1
  Signal In/1 -> Add/1
  Noise On/1 -> Switch/2
  Switch/1 -> Signal Out/1
  Signal1/1 -> Switch/3

== system HILModel/6DOF Model/Subsystem2 ==
  Signal In : Inport  Orientation=down
  Noise On : Inport  Port=2
  Add : Sum  OutScaling=2^-10
  Random Number : RandomNumber  Variance=nv  Seed=ns  SampleTime=st
  Signal1 : InportShadow  Port=1  LatchByCopyingInsideSignal=off
  Switch : Switch  Threshold=0.3
  Signal Out : Outport
  wires:
  Signal1/1 -> Switch/3
  Switch/1 -> Signal Out/1
  Noise On/1 -> Switch/2
  Signal In/1 -> Add/1
  Add/1 -> Switch/1
  Random Number/1 -> Add/2

== system HILModel/6DOF Model/Subsystem3 ==
  Signal In : Inport  Orientation=down
  Noise On : Inport  Port=2
  Add : Sum  OutScaling=2^-10
  Random Number : RandomNumber  Variance=nv  Seed=ns  SampleTime=st
  Signal1 : InportShadow  Port=1  LatchByCopyingInsideSignal=off
  Switch : Switch  Threshold=0.3
  Signal Out : Outport
  wires:
  Random Number/1 -> Add/2
  Add/1 -> Switch/1
  Signal In/1 -> Add/1
  Noise On/1 -> Switch/2
  Switch/1 -> Signal Out/1
  Signal1/1 -> Switch/3

== system HILModel/6DOF Model/Subsystem4 ==
  Signal In : Inport  Orientation=down
  Noise On : Inport  Port=2
  Add : Sum  OutScaling=2^-10
  Random Number : RandomNumber  Variance=nv  Seed=ns  SampleTime=st
  Signal1 : InportShadow  Port=1  LatchByCopyingInsideSignal=off
  Switch : Switch  Threshold=0.3
  Signal Out : Outport
  wires:
  Random Number/1 -> Add/2
  Add/1 -> Switch/1
  Signal In/1 -> Add/1
  Noise On/1 -> Switch/2
  Switch/1 -> Signal Out/1
  Signal1/1 -> Switch/3

== system HILModel/6DOF Model/Subsystem5 ==
  Signal In : Inport  Orientation=down
  Noise On : Inport  Port=2
  Add : Sum  OutScaling=2^-10
  Random Number : RandomNumber  Variance=nv  Seed=ns  SampleTime=st
  Signal1 : InportShadow  Port=1  LatchByCopyingInsideSignal=off
  Switch : Switch  Threshold=0.3
  Signal Out : Outport
  wires:
  Signal1/1 -> Switch/3
  Switch/1 -> Signal Out/1
  Noise On/1 -> Switch/2
  Signal In/1 -> Add/1
  Add/1 -> Switch/1
  Random Number/1 -> Add/2

== system HILModel/6DOF Model/Subsystem6 ==
  Signal In : Inport  Orientation=down
  Noise On : Inport  Port=2
  Add : Sum  OutScaling=2^-10
  Random Number : RandomNumber  Variance=nv  Seed=ns  SampleTime=st
  Signal1 : InportShadow  Port=1  LatchByCopyingInsideSignal=off
  Switch : Switch  Threshold=0.3
  Signal Out : Outport
  wires:
  Random Number/1 -> Add/2
  Add/1 -> Switch/1
  Signal In/1 -> Add/1
  Noise On/1 -> Switch/2
  Switch/1 -> Signal Out/1
  Signal1/1 -> Switch/3

== system HILModel/Get Delay/Detect Change ==
  Data : Inport
  Abs1 : Abs  SampleTime=SampleT
  Difference1 : simulink/Discrete/Difference  SystemSampleTime=-1  ICPrevInput=0.0  OutDataType=sfix(16)  OutScaling=2^-10  DoSatur=off
  Saturation1 : Saturate  UpperLimit=1  LowerLimit=0  SampleTime=SampleT
  change? : Outport
  wires:
  Difference1/1 -> Abs1/1
  Abs1/1 -> Saturation1/1
  Data/1 -> Difference1/1
  Saturation1/1 -> change?/1

== system HILModel/Get Delay/GPSAlive ==
  update? : Inport
  Constant : Constant
  Constant1 : Constant  Value=0
  Constant2 : Constant  Value=SampleT
  Discrete-Time Integrator : DiscreteIntegrator  ExternalReset=rising  InitialConditionSource=external  SampleTime=SampleT  ICPrevOutput=DiscIntNeverNeededParam  ICPrevScaledInput=DiscIntNeverNeededParam
  Integer Delay2 : simulink/Discrete/Integer Delay  vinit=0.0  samptime=-1  NumDelays=1
  Sum : Sum  Inputs=|++
  Update TIme : Outport
  wires:
  Constant/1 -> Discrete-Time Integrator/1
  Constant1/1 -> Discrete-Time Integrator/3
  Discrete-Time Integrator/1 -> Integer Delay2/1
  update?/1 -> Discrete-Time Integrator/2
  Integer Delay2/1 -> Sum/1
  Constant2/1 -> Sum/2
  Sum/1 -> Update TIme/1

== system HILModel/6DOF Model/Plant/6-DOF EOM ==
  "[F,M]" : Inport
  Vb Corr : Inport  Orientation=left  Port=2
  Angular Rates : Integrator  InitialCondition=PQR_0'
  Demux1 : Demux  Outputs=2
  Euler Angles : Integrator  InitialCondition=Euler_0
  Get Euler Dot : Subsystem
      mask Display:
      | port_label('input', 1, 'p, q, r')
      | port_label('input', 2, 'Euler')
      | port_label('output', 1, 'Euler_dot')
  Mux : Mux  Orientation=left  Inputs=[3;3]
  NED2NEU : Gain  Gain=[1 0 0;0 1 0;0 0 -1]  Multiplication=Matrix(K*u)  SaturateOnIntegerOverflow=on
  Position : Integrator  InitialCondition=Pos_0'
  RB2L * Vb : Product  Multiplication=Matrix(*)  SaturateOnIntegerOverflow=on  InputSameDT=on
  RB2LTP : Subsystem
  Velocities Body : Integrator  InitialCondition=Vb_0'
  "[V1,2,3,W1,2,3]" : Subsystem
  X,Y,Z (LTP) : Outport
  "Vx, Vy, Vz" : Outport  Port=2
  Euler : Outport  Port=3
  "p, q, r" : Outport  Orientation=left  Port=4
  Vb : Outport  Port=5
  Ab meas : Outport  Port=6
  Euler_dot : Outport  Port=7
  wires:
  "[V1,2,3,W1,2,3]"/1("Acc_meas ") -> Ab meas/1
  Euler Angles/1 -> "[V1,2,3,W1,2,3]"/2(Euler), Get Euler Dot/2(Euler), Euler/1, RB2LTP/1(Euler)
  Demux1/1 -> Velocities Body/1
  "[V1,2,3,W1,2,3]"/2(V*dot) -> Demux1/1
  Demux1/2 -> Angular Rates/1
  "[F,M]"/1 -> "[V1,2,3,W1,2,3]"/1("[F ; M]")
  RB2LTP/1(Rot) -> RB2L * Vb/1
  Velocities Body/1 -> Vb/1, RB2L * Vb/2
  Mux/1 -> "[V1,2,3,W1,2,3]"/3(V*)
  Position/1 -> X,Y,Z (LTP)/1
  Angular Rates/1 -> Get Euler Dot/1(p,q,r), Mux/2, "p, q, r"/1
  RB2L * Vb/1 -> NED2NEU/1, "Vx, Vy, Vz"/1  "NED"
  NED2NEU/1 -> Position/1
  Get Euler Dot/1(Euler_dot) -> Euler Angles/1, Euler_dot/1
  Vb Corr/1 -> Mux/1

== system HILModel/6DOF Model/Plant/Engine Model ==
  dt : Inport
  Vmag : Inport  Port=2
  Constant4 : Constant  Value=0
  Get To1 : Subsystem
  Mux : Mux  Inputs=2
  Mux1 : Mux  Inputs=3
  Thrust Available (lbs) : Fcn  Expr=u(1) - 0.047*sqrt(u(1))*u(2)
  kg2N : Gain  Gain=ISA_g  SaturateOnIntegerOverflow=on
  lbs2kg : Gain  Gain=0.45359237  SaturateOnIntegerOverflow=on
  Thrust : Outport
  wires:
  dt/1 -> Get To1/1(dt)
  Get To1/1(To) -> Mux/1
  Mux/1 -> Thrust Available (lbs)/1
  Thrust Available (lbs)/1 -> lbs2kg/1
  Vmag/1 -> Mux/2
  Mux1/1 -> Thrust/1
  lbs2kg/1 -> kg2N/1
  Constant4/1 -> Mux1/2, Mux1/3
  kg2N/1 -> Mux1/1

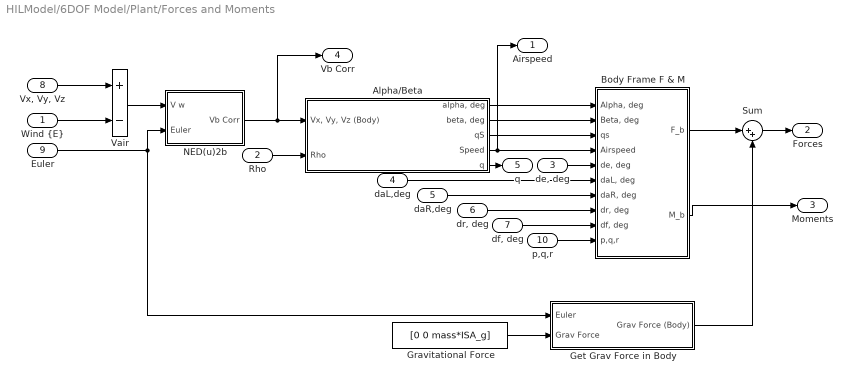
== system HILModel/6DOF Model/Plant/Forces and Moments ==
  "Wind {E}" : Inport
  Rho : Inport  Port=2
  "de, deg" : Inport  Port=3
  daL,deg : Inport  Port=4
  daR,deg : Inport  Port=5
  "dr, deg" : Inport  Port=6
  "df, deg" : Inport  Port=7
  "Vx, Vy, Vz " : Inport  Port=8
  Euler : Inport  Port=9  PortDimensions=3
  p,q,r : Inport  Port=10
  Alpha/Beta : Subsystem
  Body Frame F & M : Subsystem
  Get Grav Force in Body : Subsystem
  Gravitational Force : Constant  Value=[0 0 mass*ISA_g]  VectorParams1D=off
  NED(u)2b : Subsystem
  Sum : Sum  Inputs=|++  SaturateOnIntegerOverflow=on
  Vair : Sum  Inputs=+-  SaturateOnIntegerOverflow=on  InputSameDT=on
  Airspeed : Outport
  Forces : Outport  Port=2
  Moments : Outport  Port=3
  Vb Corr : Outport  Port=4
  q : Outport  Port=5
  wires:
  Get Grav Force in Body/1(Grav Force (Body)) -> Sum/2
  Alpha/Beta/5(q) -> q/1
  "Vx, Vy, Vz "/1 -> Vair/1
  Vair/1 -> NED(u)2b/1(V w)
  Euler/1 -> NED(u)2b/2(Euler), Get Grav Force in Body/1(Euler)
  Rho/1 -> Alpha/Beta/2(Rho)
  NED(u)2b/1(Vb Corr) -> Alpha/Beta/1("Vx, Vy, Vz (Body)"), Vb Corr/1
  Body Frame F & M/2(M_b) -> Moments/1
  Gravitational Force/1 -> Get Grav Force in Body/2(Grav Force)
  Body Frame F & M/1(F_b) -> Sum/1
  Sum/1 -> Forces/1
  Alpha/Beta/3(qS) -> Body Frame F & M/3(qs)
  Alpha/Beta/4(Speed) -> Body Frame F & M/4(Airspeed), Airspeed/1
  "df, deg"/1 -> Body Frame F & M/9("df, deg")
  p,q,r/1 -> Body Frame F & M/10(p,q,r)
  Alpha/Beta/2("beta, deg") -> Body Frame F & M/2("Beta, deg")
  "dr, deg"/1 -> Body Frame F & M/8("dr, deg")
  daL,deg/1 -> Body Frame F & M/6("daL, deg")
  Alpha/Beta/1("alpha, deg") -> Body Frame F & M/1("Alpha, deg")
  "de, deg"/1 -> Body Frame F & M/5("de, deg")
  "Wind {E}"/1 -> Vair/2
  daR,deg/1 -> Body Frame F & M/7("daR, deg")

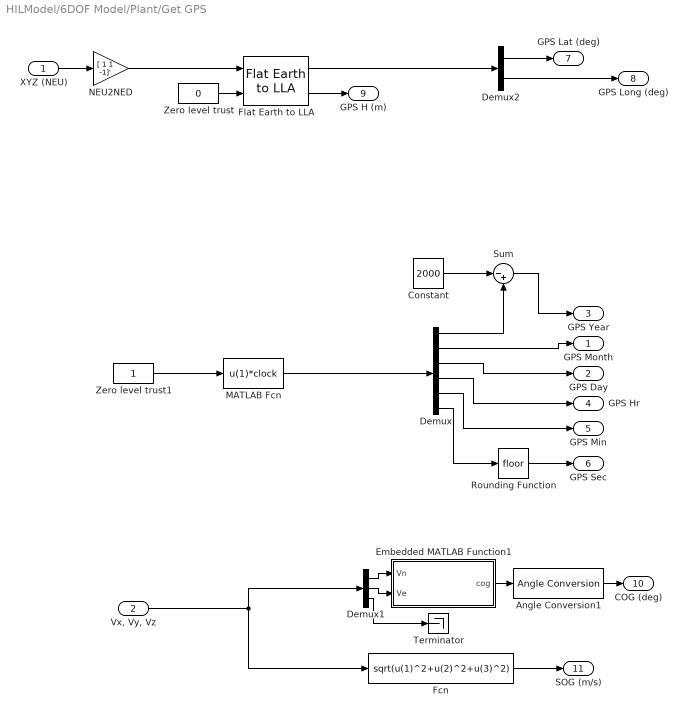
== system HILModel/6DOF Model/Plant/Get GPS ==
  XYZ (NEU) : Inport
  "Vx, Vy, Vz" : Inport  Port=2
  Angle Conversion1 : aerolibconvert2/Angle Conversion  SystemSampleTime=-1  IU=rad  OU=deg
  Constant : Constant  Value=2000
  Demux : Demux  Outputs=6
  Demux1 : Demux  Outputs=3
  Demux2 : Demux  Outputs=2
  Embedded MATLAB Function1 : Stateflow chart
  Fcn : Fcn  Expr=sqrt(u(1)^2+u(2)^2+u(3)^2)
  Flat Earth to LLA : aerolibtransform2/Flat Earth to LLA  SystemSampleTime=-1  units=Metric (MKS)  ptype=Earth (WGS84)  F=1/298.257223563  R=6378137  LL0=[GS_location(2) GS_location(3)]  psi=0
  MATLAB Fcn : MATLABFcn  MATLABFcn=u(1)*clock  OutputSignalType=real  SampleTime=SampleT
  NEU2NED : Gain  Gain=[ 1 1 -1]'  SaturateOnIntegerOverflow=on
  Rounding Function : Rounding
  Sum : Sum  Inputs=|-+
  Terminator : Terminator
  Zero level trust : Constant  Value=0  SampleTime=SampleT
  Zero level trust1 : Constant  SampleTime=SampleT
  GPS Month : Outport
  GPS Day : Outport  Port=2
  GPS Year : Outport  Port=3
  GPS Hr : Outport  Port=4
  GPS Min : Outport  Port=5
  GPS Sec : Outport  Port=6
  GPS Lat (deg) : Outport  Port=7
  GPS Long (deg) : Outport  Port=8
  GPS H (m) : Outport  Port=9
  COG (deg) : Outport  Port=10
  SOG (m/s) : Outport  Port=11
  wires:
  NEU2NED/1 -> Flat Earth to LLA/1
  Zero level trust/1 -> Flat Earth to LLA/2
  XYZ (NEU)/1 -> NEU2NED/1
  Flat Earth to LLA/1 -> Demux2/1
  Flat Earth to LLA/2 -> GPS H (m)/1
  Zero level trust1/1 -> MATLAB Fcn/1
  MATLAB Fcn/1 -> Demux/1
  Demux/2 -> GPS Month/1
  Demux/3 -> GPS Day/1
  Demux/4 -> GPS Hr/1
  Demux/5 -> GPS Min/1
  Demux/6 -> Rounding Function/1
  Rounding Function/1 -> GPS Sec/1
  Demux2/1 -> GPS Lat (deg)/1
  Demux2/2 -> GPS Long (deg)/1
  Fcn/1 -> SOG (m/s)/1
  Demux1/1 -> Embedded MATLAB Function1/1(Vn)
  Demux1/2 -> Embedded MATLAB Function1/2(Ve)
  "Vx, Vy, Vz"/1 -> Demux1/1, Fcn/1
  Embedded MATLAB Function1/1(cog) -> Angle Conversion1/1
  Angle Conversion1/1 -> COG (deg)/1
  Demux/1 -> Sum/2
  Constant/1 -> Sum/1
  Sum/1 -> GPS Year/1
  Demux1/3 -> Terminator/1

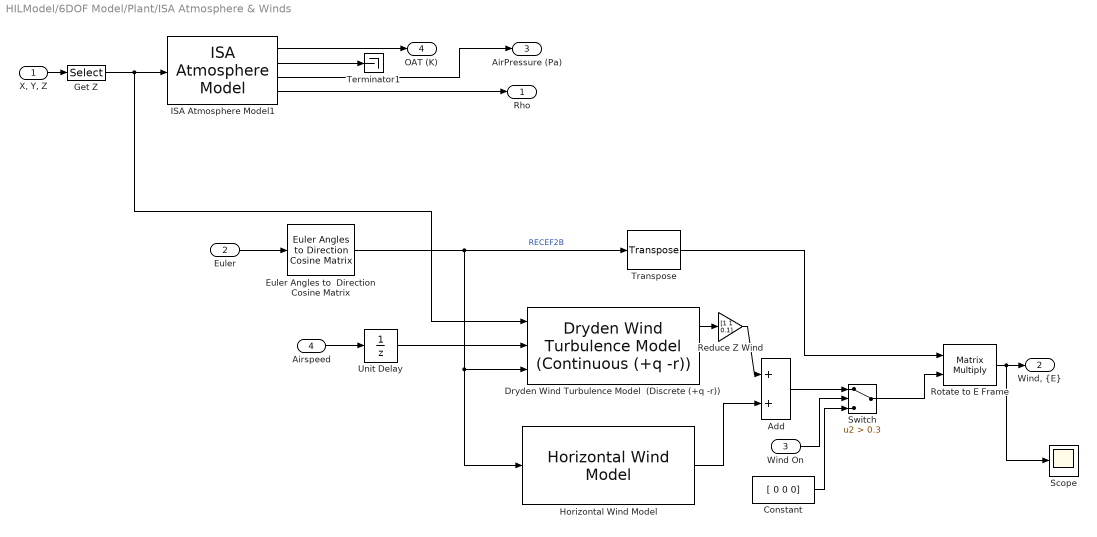
== system HILModel/6DOF Model/Plant/ISA Atmosphere & Winds ==
  "X, Y, Z" : Inport
  Euler : Inport  Port=2
  Wind On : Inport  Port=3
  Airspeed : Inport  Port=4
  Add : Sum  Inputs=2  OutScaling=2^-10
  Constant : Constant  Value=[ 0 0 0]
  Dryden Wind Turbulence Model  (Discrete (+q -r)) : aerolibwind2/Dryden Wind Turbulence Model  (Continuous (+q -r))  SystemSampleTime=-1  units=Metric (MKS)  spec=MIL-F-8785C  model=Discrete Dryden (+q -r)  W20=windBase*0.3  Wdeg=windDirTurb  TurbProb=10^-2 - Light  L_high=533.4  Wingspan=span  ts=0.005  Seed=[23341 23342 23343 23344]  T_on=on
  Euler Angles to  Direction Cosine Matrix : aerolibtransform2/Euler Angles to  Direction Cosine Matrix  SystemSampleTime=-1
  Get Z : Selector  IndexOptions=Index vector (dialog)  Indices=[3]  OutputSizes=[(-2)]  InputPortWidth=3
  Horizontal Wind Model : aerolibwind2/Horizontal Wind Model  SystemSampleTime=-1  units=Metric (MKS)  Vw_source=Internal  Vwind=windBase  W_source=Internal  Wdeg=windDirHor
  ISA Atmosphere Model1 : aerolibatmos2/ISA Atmosphere Model  SystemSampleTime=-1  custom=off  g=9.80665  gamma=1.4  R=287.0531  L=0.0065  h_trop=11000  h_strat=20000  rho0=1.225  P0=101325  T0=288.15
  Reduce Z Wind : Gain  Gain=[1 1 0.1]
  Rotate to E Frame : Product  Multiplication=Matrix(*)
  Scope : Scope
      settings: YMin=-1  YMax=13  SaveName=windData  DataFormat=Array
  Switch : Switch  Criteria=u2 > Threshold  Threshold=0.3
  Terminator1 : Terminator
  Transpose : dspmtrx3/Transpose  SystemSampleTime=-1  Hermitian=off  overflowFlag=off
  Unit Delay : UnitDelay  SampleTime=-1
  Rho : Outport
  "Wind, {E}" : Outport  Port=2
  AirPressure (Pa) : Outport  Port=3
  OAT (K) : Outport  Port=4
  wires:
  "X, Y, Z"/1 -> Get Z/1
  Get Z/1 -> ISA Atmosphere Model1/1, Dryden Wind Turbulence Model  (Discrete (+q -r))/1
  ISA Atmosphere Model1/4 -> Rho/1
  ISA Atmosphere Model1/1 -> OAT (K)/1
  ISA Atmosphere Model1/2 -> Terminator1/1
  ISA Atmosphere Model1/3 -> AirPressure (Pa)/1
  Euler/1 -> Euler Angles to  Direction Cosine Matrix/1
  Euler Angles to  Direction Cosine Matrix/1 -> Dryden Wind Turbulence Model  (Discrete (+q -r))/3, Horizontal Wind Model/1, Transpose/1  "RECEF2B"
  Airspeed/1 -> Unit Delay/1
  Add/1 -> Switch/1
  Unit Delay/1 -> Dryden Wind Turbulence Model  (Discrete (+q -r))/2
  Horizontal Wind Model/1 -> Add/2
  Switch/1 -> Rotate to E Frame/2
  Wind On/1 -> Switch/2
  Constant/1 -> Switch/3
  Transpose/1 -> Rotate to E Frame/1
  Rotate to E Frame/1 -> "Wind, {E}"/1, Scope/1
  Dryden Wind Turbulence Model  (Discrete (+q -r))/1 -> Reduce Z Wind/1
  Reduce Z Wind/1 -> Add/1

== system HILModel/6DOF Model/Plant/Magnetometer ==
  Euler : Inport
  LTP2B : dspmtrx3/Transpose  SystemSampleTime=-1  Hermitian=off  overflowFlag=off
  Mag Field in nT source:  http://www.ngdc.noaa.gov/geomagmodels/struts/calcIGRFWMM : Constant  Value=magField
  Product : Product  Multiplication=Matrix(*)  RndMeth=Zero
  RB2LTP : Subsystem
  "Mag, nT" : Outport
  wires:
  RB2LTP/1(Rot) -> LTP2B/1
  LTP2B/1 -> Product/1
  Mag Field in nT source:  http://www.ngdc.noaa.gov/geomagmodels/struts/calcIGRFWMM/1 -> Product/2
  Euler/1 -> RB2LTP/1(Euler)
  Product/1 -> "Mag, nT"/1

== system HILModel/6DOF Model/Plant/Wrap Around PSI1 ==
  Euler : Inport
  Compare To Zero : simulink/Logic and Bit Operations/Compare To Zero  SystemSampleTime=-1  relop=>=  LogicOutDataTypeMode=uint8  ZeroCross=off
  Logical Operator : Logic  Operator=NOT  AllPortsSameDT=off  OutDataTypeMode=Boolean
  Merge : Merge
  Mux2 : Mux  Inputs=2
  Negative Yaw : Subsystem
  Positive Yaw : Subsystem
  Selector1 : Selector  IndexOptions=Index vector (dialog)  Indices=[1 2]  OutputSizes=1  InputPortWidth=3
  Selector2 : Selector  IndexOptions=Index vector (dialog)  Indices=[3]  OutputSizes=1  InputPortWidth=3
  Euler-Wrapped : Outport
  wires:
  Euler/1 -> Selector2/1, Selector1/1
  Selector1/1 -> Mux2/1
  Mux2/1 -> Euler-Wrapped/1
  Selector2/1 -> Compare To Zero/1, Positive Yaw/1(yaw), Negative Yaw/1(yaw)
  Compare To Zero/1 -> Positive Yaw/Enable, Logical Operator/1
  Logical Operator/1 -> Negative Yaw/Enable
  Merge/1 -> Mux2/2
  Positive Yaw/1(yaw_wr) -> Merge/1
  Negative Yaw/1(yaw_wr) -> Merge/2

== system HILModel/6DOF Model/Split Ailerons And Introduce Failures/Aileron Flaping Failure ==
  Pulse Generator1 : DiscretePulseGenerator  PulseType=Time based  Amplitude=da_failamp  Period=da_failper  PulseWidth=50
  Vair2 : Sum  Inputs=+++  SaturateOnIntegerOverflow=on  InputSameDT=on
  da_failbias : Constant  Value=da_failbias
  da_failbias1 : Constant  Value=0
  "da, Fail, deg" : Outport
  wires:
  Vair2/1 -> "da, Fail, deg"/1
  da_failbias1/1 -> Vair2/3
  da_failbias/1 -> Vair2/2
  Pulse Generator1/1 -> Vair2/1

== system HILModel/6DOF Model/Plant/6-DOF EOM/Get Euler Dot ==
  p,q,r : Inport
  Euler : Inport  Port=2
  Mux1 : Mux  Inputs=[3 3]
  Mux2 : Mux  Inputs=3
  phidot : Fcn  Expr=u[1]+u[2]*sin(u[4])*tan(u[5])+u[3]*cos(u[4])*tan(u[5])
  psidot : Fcn  Expr=u[2]*sin(u[4])/cos(u[5])+u[3]*cos(u[4])/cos(u[5])
  thetadot : Fcn  Expr=u[2]*cos(u[4])-u[3]*sin(u[4])
  Euler_dot : Outport
  wires:
  Mux2/1 -> Euler_dot/1
  phidot/1 -> Mux2/1
  thetadot/1 -> Mux2/2
  psidot/1 -> Mux2/3
  Mux1/1 -> thetadot/1, phidot/1, psidot/1
  p,q,r/1 -> Mux1/1
  Euler/1 -> Mux1/2

== system HILModel/6DOF Model/Plant/6-DOF EOM/RB2LTP ==
  Euler : Inport
  11 : Fcn  Expr=cos(u[3])*cos(u[2])
  12 : Fcn  Expr=sin(u[3])*cos(u[2])
  13 : Fcn  Expr=-sin(u[2])
  21 : Fcn  Expr=cos(u[3])*sin(u[2])*sin(u[1])-sin(u[3])*cos(u[1])
  22 : Fcn  Expr=sin(u[3])*sin(u[2])*sin(u[1])+cos(u[3])*cos(u[1])
  23 : Fcn  Expr=cos(u[2])*sin(u[1])
  31 : Fcn  Expr=cos(u[3])*sin(u[2])*cos(u[1])+sin(u[3])*sin(u[1])
  32 : Fcn  Expr=sin(u[3])*sin(u[2])*cos(u[1])-cos(u[3])*sin(u[1])
  33 : Fcn  Expr=cos(u[2])*cos(u[1])
  Mux2 : Mux  Inputs=9
  Reshape : Reshape  OutputDimensionality=Customize  OutputDimensions=[3,3]
  Rot : Outport
  wires:
  33/1 -> Mux2/9
  32/1 -> Mux2/8
  31/1 -> Mux2/7
  23/1 -> Mux2/6
  22/1 -> Mux2/5
  21/1 -> Mux2/4
  13/1 -> Mux2/3
  12/1 -> Mux2/2
  11/1 -> Mux2/1
  Mux2/1 -> Reshape/1
  Euler/1 -> 11/1, 33/1, 32/1, 31/1, 23/1, 22/1, 21/1, 13/1, 12/1
  Reshape/1 -> Rot/1
